simulink model "gm_IP_Core_SS_Switch_and_PWM"  (R2021a)
settings: Solver=VariableStepAuto  StartTime=0.0  StopTime=0.05  RelTol=1e-3
undefined symbols (not defined in the file or in its folder): f_FPGA_clk, T_FPGA_clk
libraries: hdlsllib x1
(part 2 of 2)

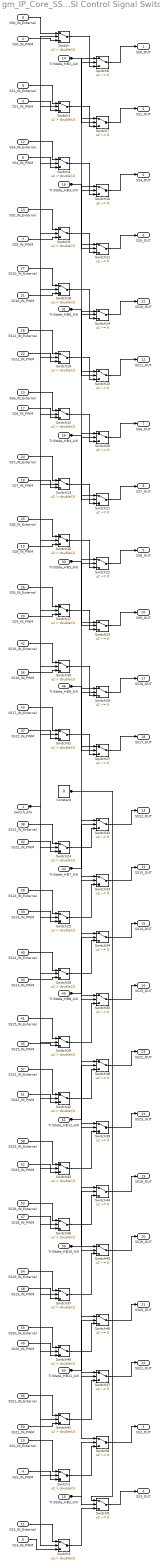
== system gm_IP_Core_SS_Switch_and_PWM/PWM_and_Switching_Signal_Control/VSI Control Signal Switch ==
  Switch_AXI : Inport  OutDataTypeStr=fixdt(0, 2, 0)  PortDimensions=1  SampleTime=1e-08
  SS0_IN_PWM : Inport  Port=2  OutDataTypeStr=fixdt(0, 1, 0)  PortDimensions=1  SampleTime=1e-08
  SS1_IN_PWM : Inport  Port=3  OutDataTypeStr=fixdt(0, 1, 0)  PortDimensions=1  SampleTime=1e-08
  SS2_IN_PWM : Inport  Port=4  OutDataTypeStr=fixdt(0, 1, 0)  PortDimensions=1  SampleTime=1e-08
  SS3_IN_PWM : Inport  Port=5  OutDataTypeStr=fixdt(0, 1, 0)  PortDimensions=1  SampleTime=1e-08
  SS4_IN_PWM : Inport  Port=6  OutDataTypeStr=fixdt(0, 1, 0)  PortDimensions=1  SampleTime=1e-08
  SS5_IN_PWM : Inport  Port=7  OutDataTypeStr=fixdt(0, 1, 0)  PortDimensions=1  SampleTime=1e-08
  SS0_IN_External : Inport  Port=8  OutDataTypeStr=boolean  PortDimensions=1  SampleTime=1e-08
  SS1_IN_External : Inport  Port=9  OutDataTypeStr=boolean  PortDimensions=1  SampleTime=1e-08
  SS2_IN_External : Inport  Port=10  OutDataTypeStr=boolean  PortDimensions=1  SampleTime=1e-08
  SS3_IN_External : Inport  Port=11  OutDataTypeStr=boolean  PortDimensions=1  SampleTime=1e-08
  SS4_IN_External : Inport  Port=12  OutDataTypeStr=boolean  PortDimensions=1  SampleTime=1e-08
  SS5_IN_External : Inport  Port=13  OutDataTypeStr=boolean  PortDimensions=1  SampleTime=1e-08
  TriState_HB1_AXI : Inport  Port=14  OutDataTypeStr=fixdt(0, 2, 0)  PortDimensions=1  SampleTime=1e-08
  TriState_HB2_AXI : Inport  Port=15  OutDataTypeStr=fixdt(0, 2, 0)  PortDimensions=1  SampleTime=1e-08
  TriState_HB3_AXI : Inport  Port=16  OutDataTypeStr=fixdt(0, 2, 0)  PortDimensions=1  SampleTime=1e-08
  SS6_IN_PWM : Inport  Port=17  OutDataTypeStr=fixdt(0, 1, 0)  PortDimensions=1  SampleTime=1e-08
  SS7_IN_PWM : Inport  Port=18  OutDataTypeStr=fixdt(0, 1, 0)  PortDimensions=1  SampleTime=1e-08
  SS8_IN_PWM : Inport  Port=19  OutDataTypeStr=fixdt(0, 1, 0)  PortDimensions=1  SampleTime=1e-08
  SS9_IN_PWM : Inport  Port=20  OutDataTypeStr=fixdt(0, 1, 0)  PortDimensions=1  SampleTime=1e-08
  SS10_IN_PWM : Inport  Port=21  OutDataTypeStr=fixdt(0, 1, 0)  PortDimensions=1  SampleTime=1e-08
  SS11_IN_PWM : Inport  Port=22  OutDataTypeStr=fixdt(0, 1, 0)  PortDimensions=1  SampleTime=1e-08
  SS6_IN_External : Inport  Port=23  OutDataTypeStr=boolean  PortDimensions=1  SampleTime=1e-08
  SS7_IN_External : Inport  Port=24  OutDataTypeStr=boolean  PortDimensions=1  SampleTime=1e-08
  SS8_IN_External : Inport  Port=25  OutDataTypeStr=boolean  PortDimensions=1  SampleTime=1e-08
  SS9_IN_External : Inport  Port=26  OutDataTypeStr=boolean  PortDimensions=1  SampleTime=1e-08
  SS10_IN_External : Inport  Port=27  OutDataTypeStr=boolean  PortDimensions=1  SampleTime=1e-08
  SS11_IN_External : Inport  Port=28  OutDataTypeStr=boolean  PortDimensions=1  SampleTime=1e-08
  TriState_HB4_AXI : Inport  Port=29  OutDataTypeStr=fixdt(0, 2, 0)  PortDimensions=1  SampleTime=1e-08
  TriState_HB5_AXI : Inport  Port=30  OutDataTypeStr=fixdt(0, 2, 0)  PortDimensions=1  SampleTime=1e-08
  TriState_HB6_AXI : Inport  Port=31  OutDataTypeStr=fixdt(0, 2, 0)  PortDimensions=1  SampleTime=1e-08
  SS12_IN_PWM : Inport  Port=32  OutDataTypeStr=fixdt(0, 1, 0)  PortDimensions=1  SampleTime=1e-08
  SS13_IN_PWM : Inport  Port=33  OutDataTypeStr=fixdt(0, 1, 0)  PortDimensions=1  SampleTime=1e-08
  SS14_IN_PWM : Inport  Port=34  OutDataTypeStr=fixdt(0, 1, 0)  PortDimensions=1  SampleTime=1e-08
  SS15_IN_PWM : Inport  Port=35  OutDataTypeStr=fixdt(0, 1, 0)  PortDimensions=1  SampleTime=1e-08
  SS16_IN_PWM : Inport  Port=36  OutDataTypeStr=fixdt(0, 1, 0)  PortDimensions=1  SampleTime=1e-08
  SS17_IN_PWM : Inport  Port=37  OutDataTypeStr=fixdt(0, 1, 0)  PortDimensions=1  SampleTime=1e-08
  SS12_IN_External : Inport  Port=38  OutDataTypeStr=boolean  PortDimensions=1  SampleTime=1e-08
  SS13_IN_External : Inport  Port=39  OutDataTypeStr=boolean  PortDimensions=1  SampleTime=1e-08
  SS14_IN_External : Inport  Port=40  OutDataTypeStr=boolean  PortDimensions=1  SampleTime=1e-08
  SS15_IN_External : Inport  Port=41  OutDataTypeStr=boolean  PortDimensions=1  SampleTime=1e-08
  SS16_IN_External : Inport  Port=42  OutDataTypeStr=boolean  PortDimensions=1  SampleTime=1e-08
  SS17_IN_External : Inport  Port=43  OutDataTypeStr=boolean  PortDimensions=1  SampleTime=1e-08
  TriState_HB7_AXI : Inport  Port=44  OutDataTypeStr=fixdt(0, 2, 0)  PortDimensions=1  SampleTime=1e-08
  TriState_HB8_AXI : Inport  Port=45  OutDataTypeStr=fixdt(0, 2, 0)  PortDimensions=1  SampleTime=1e-08
  TriState_HB9_AXI : Inport  Port=46  OutDataTypeStr=fixdt(0, 2, 0)  PortDimensions=1  SampleTime=1e-08
  SS18_IN_PWM : Inport  Port=47  OutDataTypeStr=fixdt(0, 1, 0)  PortDimensions=1  SampleTime=1e-08
  SS19_IN_PWM : Inport  Port=48  OutDataTypeStr=fixdt(0, 1, 0)  PortDimensions=1  SampleTime=1e-08
  SS20_IN_PWM : Inport  Port=49  OutDataTypeStr=fixdt(0, 1, 0)  PortDimensions=1  SampleTime=1e-08
  SS21_IN_PWM : Inport  Port=50  OutDataTypeStr=fixdt(0, 1, 0)  PortDimensions=1  SampleTime=1e-08
  SS22_IN_PWM : Inport  Port=51  OutDataTypeStr=fixdt(0, 1, 0)  PortDimensions=1  SampleTime=1e-08
  SS23_IN_PWM : Inport  Port=52  OutDataTypeStr=fixdt(0, 1, 0)  PortDimensions=1  SampleTime=1e-08
  SS18_IN_External : Inport  Port=53  OutDataTypeStr=boolean  PortDimensions=1  SampleTime=1e-08
  SS19_IN_External : Inport  Port=54  OutDataTypeStr=boolean  PortDimensions=1  SampleTime=1e-08
  SS20_IN_External : Inport  Port=55  OutDataTypeStr=boolean  PortDimensions=1  SampleTime=1e-08
  SS21_IN_External : Inport  Port=56  OutDataTypeStr=boolean  PortDimensions=1  SampleTime=1e-08
  SS22_IN_External : Inport  Port=57  OutDataTypeStr=boolean  PortDimensions=1  SampleTime=1e-08
  SS23_IN_External : Inport  Port=58  OutDataTypeStr=boolean  PortDimensions=1  SampleTime=1e-08
  TriState_HB10_AXI : Inport  Port=59  OutDataTypeStr=fixdt(0, 2, 0)  PortDimensions=1  SampleTime=1e-08
  TriState_HB11_AXI : Inport  Port=60  OutDataTypeStr=fixdt(0, 2, 0)  PortDimensions=1  SampleTime=1e-08
  TriState_HB12_AXI : Inport  Port=61  OutDataTypeStr=fixdt(0, 2, 0)  PortDimensions=1  SampleTime=1e-08
  Constant : Constant  Value=0  OutDataTypeStr=boolean  SampleTime=1e-08
  Switch{,1..5,12..13,16..19,24..25,28..31,36..37,40..43} (24 alike) : Switch  Criteria=u2 > Threshold  Threshold=double(1)  OutDataTypeStr=boolean  SampleTime=1e-08
  Switch{6..11,14..15,20..23,26..27,32..35,38..39,44..47} (24 alike) : Switch  Criteria=u2 ~= 0  Threshold=double(0)  OutDataTypeStr=boolean  SampleTime=1e-08
  SS0_OUT : Outport  SampleTime=1e-08  VectorParamsAs1DForOutWhenUnconnected=off
  SS1_OUT : Outport  Port=2  SampleTime=1e-08  VectorParamsAs1DForOutWhenUnconnected=off
  SS2_OUT : Outport  Port=3  SampleTime=1e-08  VectorParamsAs1DForOutWhenUnconnected=off
  SS3_OUT : Outport  Port=4  SampleTime=1e-08  VectorParamsAs1DForOutWhenUnconnected=off
  SS4_OUT : Outport  Port=5  SampleTime=1e-08  VectorParamsAs1DForOutWhenUnconnected=off
  SS5_OUT : Outport  Port=6  SampleTime=1e-08  VectorParamsAs1DForOutWhenUnconnected=off
  SS6_OUT : Outport  Port=7  SampleTime=1e-08  VectorParamsAs1DForOutWhenUnconnected=off
  SS7_OUT : Outport  Port=8  SampleTime=1e-08  VectorParamsAs1DForOutWhenUnconnected=off
  SS8_OUT : Outport  Port=9  SampleTime=1e-08  VectorParamsAs1DForOutWhenUnconnected=off
  SS9_OUT : Outport  Port=10  SampleTime=1e-08  VectorParamsAs1DForOutWhenUnconnected=off
  SS10_OUT : Outport  Port=11  SampleTime=1e-08  VectorParamsAs1DForOutWhenUnconnected=off
  SS11_OUT : Outport  Port=12  SampleTime=1e-08  VectorParamsAs1DForOutWhenUnconnected=off
  SS12_OUT : Outport  Port=13  SampleTime=1e-08  VectorParamsAs1DForOutWhenUnconnected=off
  SS13_OUT : Outport  Port=14  SampleTime=1e-08  VectorParamsAs1DForOutWhenUnconnected=off
  SS14_OUT : Outport  Port=15  SampleTime=1e-08  VectorParamsAs1DForOutWhenUnconnected=off
  SS15_OUT : Outport  Port=16  SampleTime=1e-08  VectorParamsAs1DForOutWhenUnconnected=off
  SS16_OUT : Outport  Port=17  SampleTime=1e-08  VectorParamsAs1DForOutWhenUnconnected=off
  SS17_OUT : Outport  Port=18  SampleTime=1e-08  VectorParamsAs1DForOutWhenUnconnected=off
  SS18_OUT : Outport  Port=19  SampleTime=1e-08  VectorParamsAs1DForOutWhenUnconnected=off
  SS19_OUT : Outport  Port=20  SampleTime=1e-08  VectorParamsAs1DForOutWhenUnconnected=off
  SS20_OUT : Outport  Port=21  SampleTime=1e-08  VectorParamsAs1DForOutWhenUnconnected=off
  SS21_OUT : Outport  Port=22  SampleTime=1e-08  VectorParamsAs1DForOutWhenUnconnected=off
  SS22_OUT : Outport  Port=23  SampleTime=1e-08  VectorParamsAs1DForOutWhenUnconnected=off
  SS23_OUT : Outport  Port=24  SampleTime=1e-08  VectorParamsAs1DForOutWhenUnconnected=off
  wires:
  Switch_AXI/1 -> Switch5/2, Switch43/2, Switch42/2, Switch41/2, Switch40/2, Switch4/2, Switch37/2, Switch36/2, Switch31/2, Switch30/2, Switch3/2, Switch29/2, Switch28/2, Switch25/2, Switch24/2, Switch2/2, Switch19/2, Switch18/2, Switch17/2, Switch16/2, Switch13/2, Switch12/2, Switch1/2, Switch/2
  SS0_IN_PWM/1 -> Switch/3
  SS1_IN_PWM/1 -> Switch1/3
  SS2_IN_PWM/1 -> Switch2/3
  SS3_IN_PWM/1 -> Switch3/3
  SS4_IN_PWM/1 -> Switch4/3
  SS5_IN_PWM/1 -> Switch5/3
  SS0_IN_External/1 -> Switch/1
  SS1_IN_External/1 -> Switch1/1
  SS2_IN_External/1 -> Switch2/1
  SS3_IN_External/1 -> Switch3/1
  SS4_IN_External/1 -> Switch4/1
  SS5_IN_External/1 -> Switch5/1
  TriState_HB1_AXI/1 -> Switch7/2, Switch6/2
  TriState_HB2_AXI/1 -> Switch9/2, Switch8/2
  TriState_HB3_AXI/1 -> Switch11/2, Switch10/2
  SS6_IN_PWM/1 -> Switch12/3
  SS7_IN_PWM/1 -> Switch13/3
  SS8_IN_PWM/1 -> Switch16/3
  SS9_IN_PWM/1 -> Switch17/3
  SS10_IN_PWM/1 -> Switch18/3
  SS11_IN_PWM/1 -> Switch19/3
  SS6_IN_External/1 -> Switch12/1
  SS7_IN_External/1 -> Switch13/1
  SS8_IN_External/1 -> Switch16/1
  SS9_IN_External/1 -> Switch17/1
  SS10_IN_External/1 -> Switch18/1
  SS11_IN_External/1 -> Switch19/1
  TriState_HB4_AXI/1 -> Switch21/2, Switch20/2
  TriState_HB5_AXI/1 -> Switch23/2, Switch22/2
  TriState_HB6_AXI/1 -> Switch15/2, Switch14/2
  SS12_IN_PWM/1 -> Switch24/3
  SS13_IN_PWM/1 -> Switch25/3
  SS14_IN_PWM/1 -> Switch28/3
  SS15_IN_PWM/1 -> Switch29/3
  SS16_IN_PWM/1 -> Switch30/3
  SS17_IN_PWM/1 -> Switch31/3
  SS12_IN_External/1 -> Switch24/1
  SS13_IN_External/1 -> Switch25/1
  SS14_IN_External/1 -> Switch28/1
  SS15_IN_External/1 -> Switch29/1
  SS16_IN_External/1 -> Switch30/1
  SS17_IN_External/1 -> Switch31/1
  TriState_HB7_AXI/1 -> Switch33/2, Switch32/2
  TriState_HB8_AXI/1 -> Switch35/2, Switch34/2
  TriState_HB9_AXI/1 -> Switch27/2, Switch26/2
  SS18_IN_PWM/1 -> Switch36/3
  SS19_IN_PWM/1 -> Switch37/3
  SS20_IN_PWM/1 -> Switch40/3
  SS21_IN_PWM/1 -> Switch41/3
  SS22_IN_PWM/1 -> Switch42/3
  SS23_IN_PWM/1 -> Switch43/3
  SS18_IN_External/1 -> Switch36/1
  SS19_IN_External/1 -> Switch37/1
  SS20_IN_External/1 -> Switch40/1
  SS21_IN_External/1 -> Switch41/1
  SS22_IN_External/1 -> Switch42/1
  SS23_IN_External/1 -> Switch43/1
  TriState_HB10_AXI/1 -> Switch45/2, Switch44/2
  TriState_HB11_AXI/1 -> Switch47/2, Switch46/2
  TriState_HB12_AXI/1 -> Switch39/2, Switch38/2
  Constant/1 -> Switch9/1, Switch8/1, Switch7/1, Switch6/1, Switch47/1, Switch46/1, Switch45/1, Switch44/1, Switch39/1, Switch38/1, Switch35/1, Switch34/1, Switch33/1, Switch32/1, Switch27/1, Switch26/1, Switch23/1, Switch22/1, Switch21/1, Switch20/1, Switch15/1, Switch14/1, Switch11/1, Switch10/1
  Switch/1 -> Switch6/3
  Switch1/1 -> Switch7/3
  Switch10/1 -> SS4_OUT/1
  Switch11/1 -> SS5_OUT/1
  Switch12/1 -> Switch20/3
  Switch13/1 -> Switch21/3
  Switch14/1 -> SS10_OUT/1
  Switch15/1 -> SS11_OUT/1
  Switch16/1 -> Switch22/3
  Switch17/1 -> Switch23/3
  Switch18/1 -> Switch14/3
  Switch19/1 -> Switch15/3
  Switch2/1 -> Switch8/3
  Switch20/1 -> SS6_OUT/1
  Switch21/1 -> SS7_OUT/1
  Switch22/1 -> SS8_OUT/1
  Switch23/1 -> SS9_OUT/1
  Switch24/1 -> Switch32/3
  Switch25/1 -> Switch33/3
  Switch26/1 -> SS16_OUT/1
  Switch27/1 -> SS17_OUT/1
  Switch28/1 -> Switch34/3
  Switch29/1 -> Switch35/3
  Switch3/1 -> Switch9/3
  Switch30/1 -> Switch26/3
  Switch31/1 -> Switch27/3
  Switch32/1 -> SS12_OUT/1
  Switch33/1 -> SS13_OUT/1
  Switch34/1 -> SS14_OUT/1
  Switch35/1 -> SS15_OUT/1
  Switch36/1 -> Switch44/3
  Switch37/1 -> Switch45/3
  Switch38/1 -> SS22_OUT/1
  Switch39/1 -> SS23_OUT/1
  Switch4/1 -> Switch10/3
  Switch40/1 -> Switch46/3
  Switch41/1 -> Switch47/3
  Switch42/1 -> Switch38/3
  Switch43/1 -> Switch39/3
  Switch44/1 -> SS18_OUT/1
  Switch45/1 -> SS19_OUT/1
  Switch46/1 -> SS20_OUT/1
  Switch47/1 -> SS21_OUT/1
  Switch5/1 -> Switch11/3
  Switch6/1 -> SS0_OUT/1
  Switch7/1 -> SS1_OUT/1
  Switch8/1 -> SS2_OUT/1
  Switch9/1 -> SS3_OUT/1

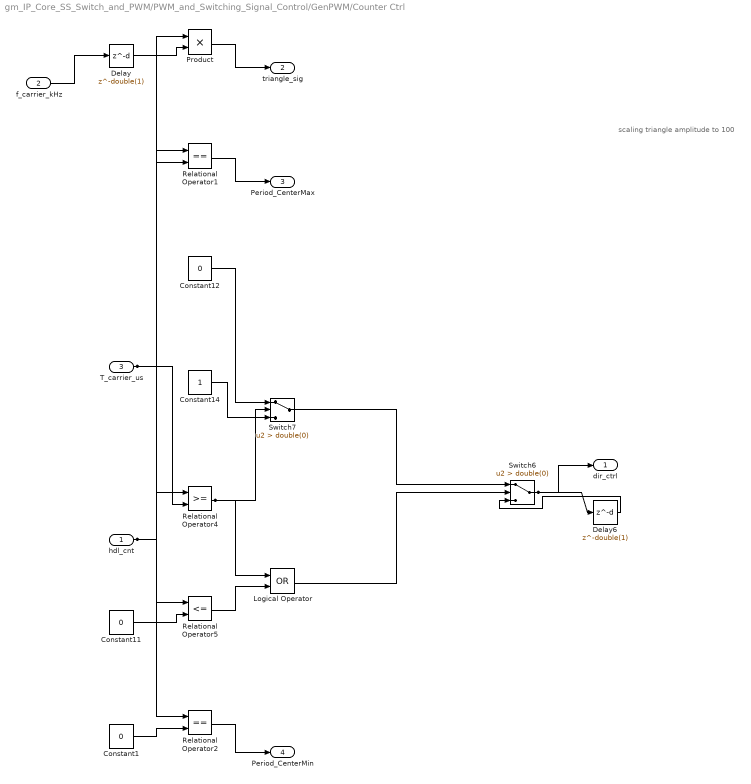
== system gm_IP_Core_SS_Switch_and_PWM/PWM_and_Switching_Signal_Control/GenPWM/Counter Ctrl ==
  note: scaling triangle amplitude to 100
  hdl_cnt : Inport  OutDataTypeStr=fixdt(0, 20, 0)  PortDimensions=1  SampleTime=1e-08
  f_carrier_kHz : Inport  Port=2  OutDataTypeStr=fixdt(0, 25, 26)  PortDimensions=1  SampleTime=1e-08
  T_carrier_us : Inport  Port=3  OutDataTypeStr=fixdt(0, 25, 0)  PortDimensions=1  SampleTime=1e-08
  Constant1 : Constant  Value=0  OutDataTypeStr=fixdt(0, 20, 0)  SampleTime=1e-08
  Constant11 : Constant  Value=0  OutDataTypeStr=fixdt(0, 20, 0)  SampleTime=1e-08
  Constant12 : Constant  Value=0  OutDataTypeStr=boolean  SampleTime=1e-08
  Constant14 : Constant  OutDataTypeStr=boolean  SampleTime=1e-08
  Delay : Delay  DelayLength=double(1)  InitialCondition=0  SampleTime=1e-08
  Delay6 : Delay  DelayLength=double(1)  InitialCondition=0  SampleTime=1e-08
  Logical Operator : Logic  Operator=OR  AllPortsSameDT=off  OutDataTypeStr=boolean  SampleTime=1e-08
  Product : Product  Inputs=**  OutDataTypeStr=fixdt(0, 18, 17)  SampleTime=1e-08
  Relational Operator1 : RelationalOperator  Operator===  OutDataTypeStr=boolean  SampleTime=1e-08  RndMeth=Nearest
  Relational Operator2 : RelationalOperator  Operator===  OutDataTypeStr=boolean  SampleTime=1e-08  RndMeth=Nearest
  Relational Operator4 : RelationalOperator  OutDataTypeStr=boolean  SampleTime=1e-08  RndMeth=Nearest
  Relational Operator5 : RelationalOperator  Operator=<=  OutDataTypeStr=boolean  SampleTime=1e-08  RndMeth=Nearest
  Switch6 : Switch  Criteria=u2 > Threshold  Threshold=double(0)  OutDataTypeStr=boolean  SampleTime=1e-08
  Switch7 : Switch  Criteria=u2 > Threshold  Threshold=double(0)  OutDataTypeStr=boolean  SampleTime=1e-08
  dir_ctrl : Outport  SampleTime=1e-08  VectorParamsAs1DForOutWhenUnconnected=off
  triangle_sig : Outport  Port=2  SampleTime=1e-08  VectorParamsAs1DForOutWhenUnconnected=off
  Period_CenterMax : Outport  Port=3  SampleTime=1e-08  VectorParamsAs1DForOutWhenUnconnected=off
  Period_CenterMin : Outport  Port=4  SampleTime=1e-08  VectorParamsAs1DForOutWhenUnconnected=off
  wires:
  hdl_cnt/1 -> Relational Operator5/1, Relational Operator4/1, Relational Operator2/1, Relational Operator1/1, Product/1
  f_carrier_kHz/1 -> Delay/1
  T_carrier_us/1 -> Relational Operator4/2, Relational Operator1/2
  Constant1/1 -> Relational Operator2/2
  Constant11/1 -> Relational Operator5/2
  Constant12/1 -> Switch7/1
  Constant14/1 -> Switch7/3
  Delay/1 -> Product/2
  Delay6/1 -> Switch6/3
  Logical Operator/1 -> Switch6/2
  Product/1 -> triangle_sig/1
  Relational Operator1/1 -> Period_CenterMax/1
  Relational Operator2/1 -> Period_CenterMin/1
  Relational Operator4/1 -> Switch7/2, Logical Operator/1
  Relational Operator5/1 -> Logical Operator/2
  Switch6/1 -> Delay6/1, dir_ctrl/1
  Switch7/1 -> Switch6/1

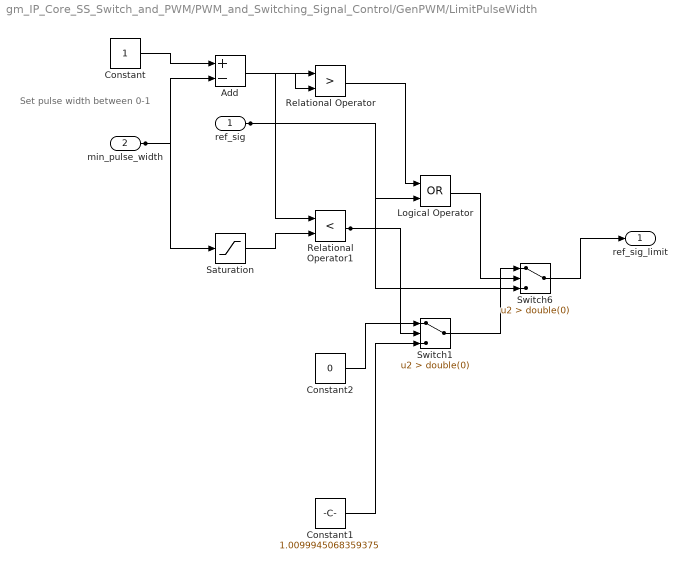
== system gm_IP_Core_SS_Switch_and_PWM/PWM_and_Switching_Signal_Control/GenPWM/LimitPulseWidth ==
  note: Set pulse width between 0-1
  ref_sig : Inport  OutDataTypeStr=fixdt(1, 14, 12)  PortDimensions=1  SampleTime=1e-08
  min_pulse_width : Inport  Port=2  OutDataTypeStr=fixdt(1, 18, 16)  PortDimensions=1  SampleTime=1e-08
  Add : Sum  Inputs=+-  AccumDataTypeStr=fixdt(1, 19, 16)  OutDataTypeStr=fixdt(1, 18, 16)  SampleTime=1e-08
  Constant : Constant  OutDataTypeStr=fixdt(1, 18, 16)  SampleTime=1e-08
  Constant1 : Constant  Value=1.0099945068359375  OutDataTypeStr=fixdt(1, 18, 16)  SampleTime=1e-08
  Constant2 : Constant  Value=0  OutDataTypeStr=fixdt(1, 18, 16)  SampleTime=1e-08
  Logical Operator : Logic  Operator=OR  AllPortsSameDT=off  OutDataTypeStr=boolean  SampleTime=1e-08
  Relational Operator : RelationalOperator  Operator=>  OutDataTypeStr=boolean  SampleTime=1e-08  RndMeth=Nearest
  Relational Operator1 : RelationalOperator  Operator=<  OutDataTypeStr=boolean  SampleTime=1e-08  RndMeth=Nearest
  Saturation : Saturate  UpperLimit="fi(0,1,18,16,\"hex\",\"10000\")"  LowerLimit="fi(0,1,18,16,\"hex\",\"00000\")"  SampleTime=1e-08  OutDataTypeStr=fixdt(1, 18, 16)
  Switch1 : Switch  Criteria=u2 > Threshold  Threshold=double(0)  OutDataTypeStr=fixdt(1, 18, 16)  SampleTime=1e-08
  Switch6 : Switch  Criteria=u2 > Threshold  Threshold=double(0)  OutDataTypeStr=fixdt(1, 18, 16)  SampleTime=1e-08
  ref_sig_limit : Outport  SampleTime=1e-08  VectorParamsAs1DForOutWhenUnconnected=off
  wires:
  ref_sig/1 -> Switch6/3, Relational Operator1/1, Relational Operator/1
  min_pulse_width/1 -> Saturation/1, Add/2
  Add/1 -> Relational Operator/2
  Constant/1 -> Add/1
  Constant1/1 -> Switch1/3
  Constant2/1 -> Switch1/1
  Logical Operator/1 -> Switch6/2
  Relational Operator/1 -> Logical Operator/1
  Relational Operator1/1 -> Switch1/2, Logical Operator/2
  Saturation/1 -> Relational Operator1/2
  Switch1/1 -> Switch6/1
  Switch6/1 -> ref_sig_limit/1

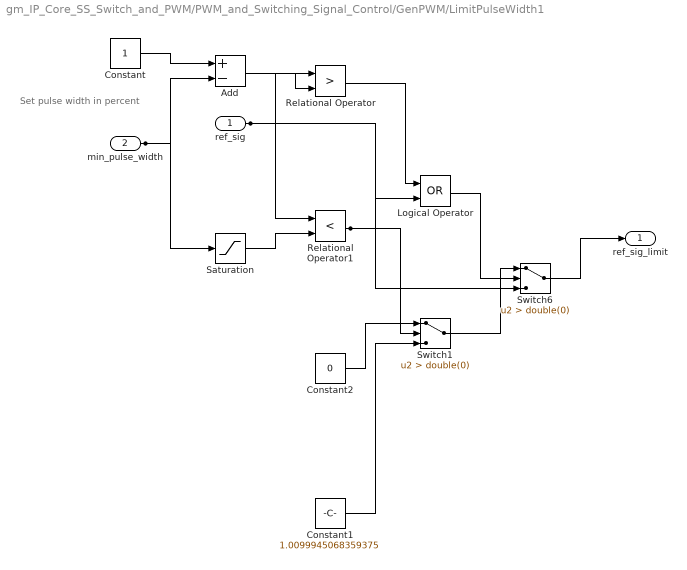
== system gm_IP_Core_SS_Switch_and_PWM/PWM_and_Switching_Signal_Control/GenPWM/LimitPulseWidth1 ==
  note: Set pulse width in percent
  ref_sig : Inport  OutDataTypeStr=fixdt(1, 14, 12)  PortDimensions=1  SampleTime=1e-08
  min_pulse_width : Inport  Port=2  OutDataTypeStr=fixdt(1, 18, 16)  PortDimensions=1  SampleTime=1e-08
  Add : Sum  Inputs=+-  AccumDataTypeStr=fixdt(1, 19, 16)  OutDataTypeStr=fixdt(1, 18, 16)  SampleTime=1e-08
  Constant : Constant  OutDataTypeStr=fixdt(1, 18, 16)  SampleTime=1e-08
  Constant1 : Constant  Value=1.0099945068359375  OutDataTypeStr=fixdt(1, 18, 16)  SampleTime=1e-08
  Constant2 : Constant  Value=0  OutDataTypeStr=fixdt(1, 18, 16)  SampleTime=1e-08
  Logical Operator : Logic  Operator=OR  AllPortsSameDT=off  OutDataTypeStr=boolean  SampleTime=1e-08
  Relational Operator : RelationalOperator  Operator=>  OutDataTypeStr=boolean  SampleTime=1e-08  RndMeth=Nearest
  Relational Operator1 : RelationalOperator  Operator=<  OutDataTypeStr=boolean  SampleTime=1e-08  RndMeth=Nearest
  Saturation : Saturate  UpperLimit="fi(0,1,18,16,\"hex\",\"10000\")"  LowerLimit="fi(0,1,18,16,\"hex\",\"00000\")"  SampleTime=1e-08  OutDataTypeStr=fixdt(1, 18, 16)
  Switch1 : Switch  Criteria=u2 > Threshold  Threshold=double(0)  OutDataTypeStr=fixdt(1, 18, 16)  SampleTime=1e-08
  Switch6 : Switch  Criteria=u2 > Threshold  Threshold=double(0)  OutDataTypeStr=fixdt(1, 18, 16)  SampleTime=1e-08
  ref_sig_limit : Outport  SampleTime=1e-08  VectorParamsAs1DForOutWhenUnconnected=off
  wires:
  ref_sig/1 -> Switch6/3, Relational Operator1/1, Relational Operator/1
  min_pulse_width/1 -> Saturation/1, Add/2
  Add/1 -> Relational Operator/2
  Constant/1 -> Add/1
  Constant1/1 -> Switch1/3
  Constant2/1 -> Switch1/1
  Logical Operator/1 -> Switch6/2
  Relational Operator/1 -> Logical Operator/1
  Relational Operator1/1 -> Switch1/2, Logical Operator/2
  Saturation/1 -> Relational Operator1/2
  Switch1/1 -> Switch6/1
  Switch6/1 -> ref_sig_limit/1

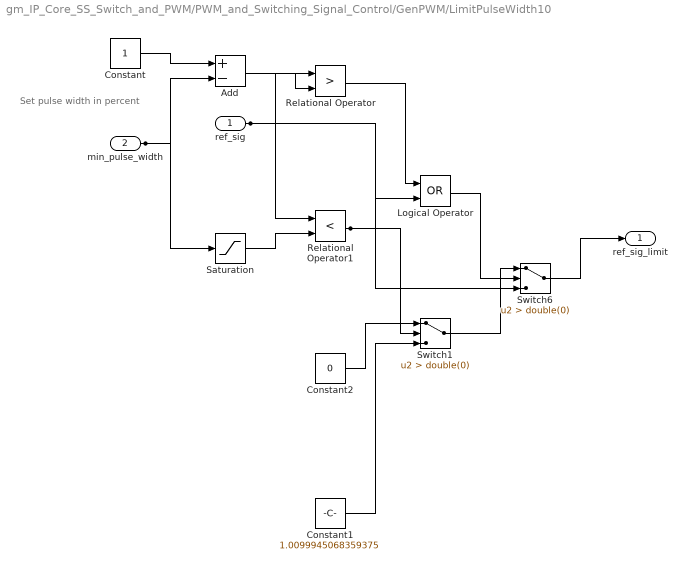
== system gm_IP_Core_SS_Switch_and_PWM/PWM_and_Switching_Signal_Control/GenPWM/LimitPulseWidth10 ==
  note: Set pulse width in percent
  ref_sig : Inport  OutDataTypeStr=fixdt(1, 14, 12)  PortDimensions=1  SampleTime=1e-08
  min_pulse_width : Inport  Port=2  OutDataTypeStr=fixdt(1, 18, 16)  PortDimensions=1  SampleTime=1e-08
  Add : Sum  Inputs=+-  AccumDataTypeStr=fixdt(1, 19, 16)  OutDataTypeStr=fixdt(1, 18, 16)  SampleTime=1e-08
  Constant : Constant  OutDataTypeStr=fixdt(1, 18, 16)  SampleTime=1e-08
  Constant1 : Constant  Value=1.0099945068359375  OutDataTypeStr=fixdt(1, 18, 16)  SampleTime=1e-08
  Constant2 : Constant  Value=0  OutDataTypeStr=fixdt(1, 18, 16)  SampleTime=1e-08
  Logical Operator : Logic  Operator=OR  AllPortsSameDT=off  OutDataTypeStr=boolean  SampleTime=1e-08
  Relational Operator : RelationalOperator  Operator=>  OutDataTypeStr=boolean  SampleTime=1e-08  RndMeth=Nearest
  Relational Operator1 : RelationalOperator  Operator=<  OutDataTypeStr=boolean  SampleTime=1e-08  RndMeth=Nearest
  Saturation : Saturate  UpperLimit="fi(0,1,18,16,\"hex\",\"10000\")"  LowerLimit="fi(0,1,18,16,\"hex\",\"00000\")"  SampleTime=1e-08  OutDataTypeStr=fixdt(1, 18, 16)
  Switch1 : Switch  Criteria=u2 > Threshold  Threshold=double(0)  OutDataTypeStr=fixdt(1, 18, 16)  SampleTime=1e-08
  Switch6 : Switch  Criteria=u2 > Threshold  Threshold=double(0)  OutDataTypeStr=fixdt(1, 18, 16)  SampleTime=1e-08
  ref_sig_limit : Outport  SampleTime=1e-08  VectorParamsAs1DForOutWhenUnconnected=off
  wires:
  ref_sig/1 -> Switch6/3, Relational Operator1/1, Relational Operator/1
  min_pulse_width/1 -> Saturation/1, Add/2
  Add/1 -> Relational Operator/2
  Constant/1 -> Add/1
  Constant1/1 -> Switch1/3
  Constant2/1 -> Switch1/1
  Logical Operator/1 -> Switch6/2
  Relational Operator/1 -> Logical Operator/1
  Relational Operator1/1 -> Switch1/2, Logical Operator/2
  Saturation/1 -> Relational Operator1/2
  Switch1/1 -> Switch6/1
  Switch6/1 -> ref_sig_limit/1

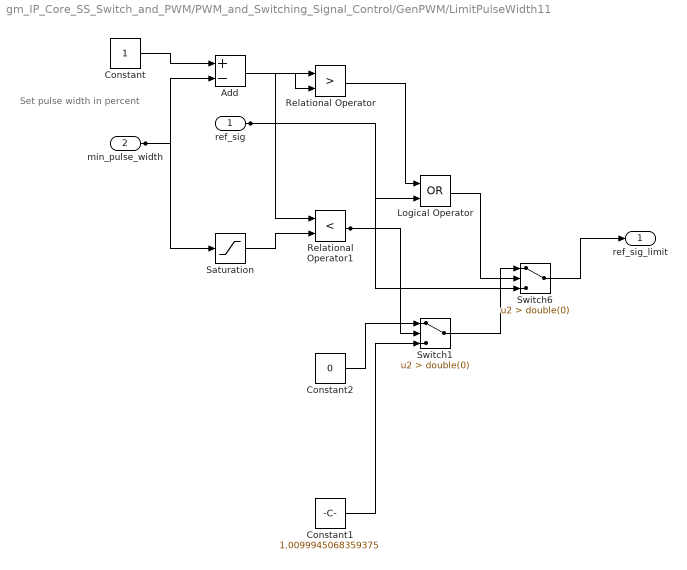
== system gm_IP_Core_SS_Switch_and_PWM/PWM_and_Switching_Signal_Control/GenPWM/LimitPulseWidth11 ==
  note: Set pulse width in percent
  ref_sig : Inport  OutDataTypeStr=fixdt(1, 14, 12)  PortDimensions=1  SampleTime=1e-08
  min_pulse_width : Inport  Port=2  OutDataTypeStr=fixdt(1, 18, 16)  PortDimensions=1  SampleTime=1e-08
  Add : Sum  Inputs=+-  AccumDataTypeStr=fixdt(1, 19, 16)  OutDataTypeStr=fixdt(1, 18, 16)  SampleTime=1e-08
  Constant : Constant  OutDataTypeStr=fixdt(1, 18, 16)  SampleTime=1e-08
  Constant1 : Constant  Value=1.0099945068359375  OutDataTypeStr=fixdt(1, 18, 16)  SampleTime=1e-08
  Constant2 : Constant  Value=0  OutDataTypeStr=fixdt(1, 18, 16)  SampleTime=1e-08
  Logical Operator : Logic  Operator=OR  AllPortsSameDT=off  OutDataTypeStr=boolean  SampleTime=1e-08
  Relational Operator : RelationalOperator  Operator=>  OutDataTypeStr=boolean  SampleTime=1e-08  RndMeth=Nearest
  Relational Operator1 : RelationalOperator  Operator=<  OutDataTypeStr=boolean  SampleTime=1e-08  RndMeth=Nearest
  Saturation : Saturate  UpperLimit="fi(0,1,18,16,\"hex\",\"10000\")"  LowerLimit="fi(0,1,18,16,\"hex\",\"00000\")"  SampleTime=1e-08  OutDataTypeStr=fixdt(1, 18, 16)
  Switch1 : Switch  Criteria=u2 > Threshold  Threshold=double(0)  OutDataTypeStr=fixdt(1, 18, 16)  SampleTime=1e-08
  Switch6 : Switch  Criteria=u2 > Threshold  Threshold=double(0)  OutDataTypeStr=fixdt(1, 18, 16)  SampleTime=1e-08
  ref_sig_limit : Outport  SampleTime=1e-08  VectorParamsAs1DForOutWhenUnconnected=off
  wires:
  ref_sig/1 -> Switch6/3, Relational Operator1/1, Relational Operator/1
  min_pulse_width/1 -> Saturation/1, Add/2
  Add/1 -> Relational Operator/2
  Constant/1 -> Add/1
  Constant1/1 -> Switch1/3
  Constant2/1 -> Switch1/1
  Logical Operator/1 -> Switch6/2
  Relational Operator/1 -> Logical Operator/1
  Relational Operator1/1 -> Switch1/2, Logical Operator/2
  Saturation/1 -> Relational Operator1/2
  Switch1/1 -> Switch6/1
  Switch6/1 -> ref_sig_limit/1

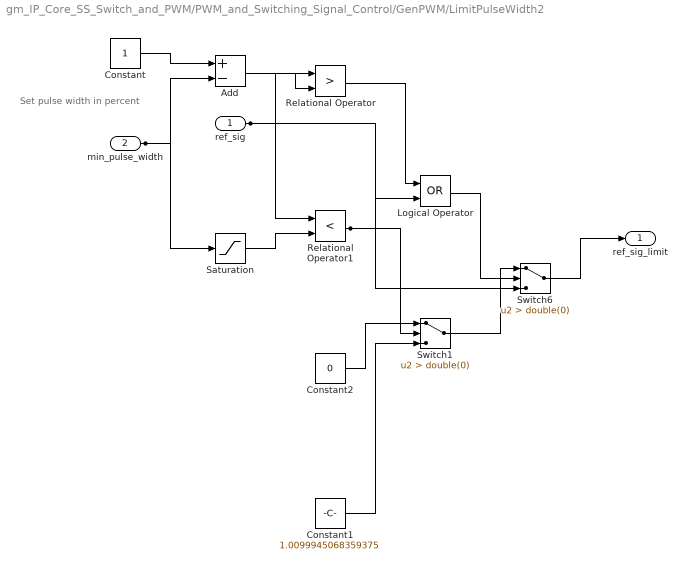
== system gm_IP_Core_SS_Switch_and_PWM/PWM_and_Switching_Signal_Control/GenPWM/LimitPulseWidth2 ==
  note: Set pulse width in percent
  ref_sig : Inport  OutDataTypeStr=fixdt(1, 14, 12)  PortDimensions=1  SampleTime=1e-08
  min_pulse_width : Inport  Port=2  OutDataTypeStr=fixdt(1, 18, 16)  PortDimensions=1  SampleTime=1e-08
  Add : Sum  Inputs=+-  AccumDataTypeStr=fixdt(1, 19, 16)  OutDataTypeStr=fixdt(1, 18, 16)  SampleTime=1e-08
  Constant : Constant  OutDataTypeStr=fixdt(1, 18, 16)  SampleTime=1e-08
  Constant1 : Constant  Value=1.0099945068359375  OutDataTypeStr=fixdt(1, 18, 16)  SampleTime=1e-08
  Constant2 : Constant  Value=0  OutDataTypeStr=fixdt(1, 18, 16)  SampleTime=1e-08
  Logical Operator : Logic  Operator=OR  AllPortsSameDT=off  OutDataTypeStr=boolean  SampleTime=1e-08
  Relational Operator : RelationalOperator  Operator=>  OutDataTypeStr=boolean  SampleTime=1e-08  RndMeth=Nearest
  Relational Operator1 : RelationalOperator  Operator=<  OutDataTypeStr=boolean  SampleTime=1e-08  RndMeth=Nearest
  Saturation : Saturate  UpperLimit="fi(0,1,18,16,\"hex\",\"10000\")"  LowerLimit="fi(0,1,18,16,\"hex\",\"00000\")"  SampleTime=1e-08  OutDataTypeStr=fixdt(1, 18, 16)
  Switch1 : Switch  Criteria=u2 > Threshold  Threshold=double(0)  OutDataTypeStr=fixdt(1, 18, 16)  SampleTime=1e-08
  Switch6 : Switch  Criteria=u2 > Threshold  Threshold=double(0)  OutDataTypeStr=fixdt(1, 18, 16)  SampleTime=1e-08
  ref_sig_limit : Outport  SampleTime=1e-08  VectorParamsAs1DForOutWhenUnconnected=off
  wires:
  ref_sig/1 -> Switch6/3, Relational Operator1/1, Relational Operator/1
  min_pulse_width/1 -> Saturation/1, Add/2
  Add/1 -> Relational Operator/2
  Constant/1 -> Add/1
  Constant1/1 -> Switch1/3
  Constant2/1 -> Switch1/1
  Logical Operator/1 -> Switch6/2
  Relational Operator/1 -> Logical Operator/1
  Relational Operator1/1 -> Switch1/2, Logical Operator/2
  Saturation/1 -> Relational Operator1/2
  Switch1/1 -> Switch6/1
  Switch6/1 -> ref_sig_limit/1

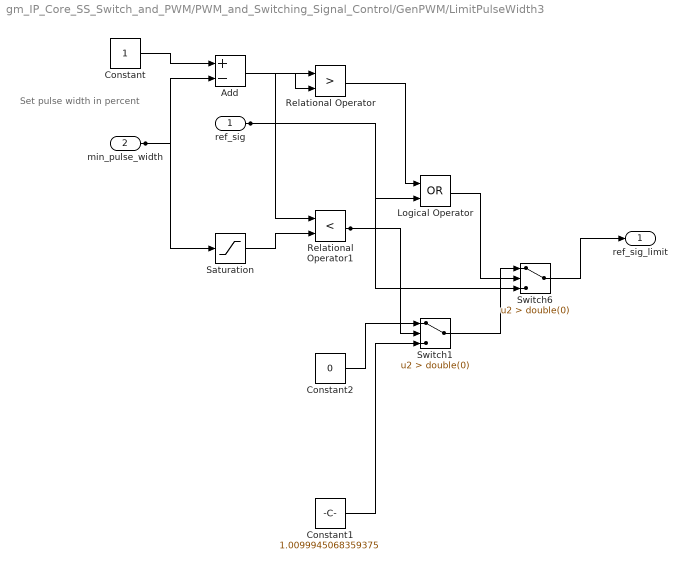
== system gm_IP_Core_SS_Switch_and_PWM/PWM_and_Switching_Signal_Control/GenPWM/LimitPulseWidth3 ==
  note: Set pulse width in percent
  ref_sig : Inport  OutDataTypeStr=fixdt(1, 14, 12)  PortDimensions=1  SampleTime=1e-08
  min_pulse_width : Inport  Port=2  OutDataTypeStr=fixdt(1, 18, 16)  PortDimensions=1  SampleTime=1e-08
  Add : Sum  Inputs=+-  AccumDataTypeStr=fixdt(1, 19, 16)  OutDataTypeStr=fixdt(1, 18, 16)  SampleTime=1e-08
  Constant : Constant  OutDataTypeStr=fixdt(1, 18, 16)  SampleTime=1e-08
  Constant1 : Constant  Value=1.0099945068359375  OutDataTypeStr=fixdt(1, 18, 16)  SampleTime=1e-08
  Constant2 : Constant  Value=0  OutDataTypeStr=fixdt(1, 18, 16)  SampleTime=1e-08
  Logical Operator : Logic  Operator=OR  AllPortsSameDT=off  OutDataTypeStr=boolean  SampleTime=1e-08
  Relational Operator : RelationalOperator  Operator=>  OutDataTypeStr=boolean  SampleTime=1e-08  RndMeth=Nearest
  Relational Operator1 : RelationalOperator  Operator=<  OutDataTypeStr=boolean  SampleTime=1e-08  RndMeth=Nearest
  Saturation : Saturate  UpperLimit="fi(0,1,18,16,\"hex\",\"10000\")"  LowerLimit="fi(0,1,18,16,\"hex\",\"00000\")"  SampleTime=1e-08  OutDataTypeStr=fixdt(1, 18, 16)
  Switch1 : Switch  Criteria=u2 > Threshold  Threshold=double(0)  OutDataTypeStr=fixdt(1, 18, 16)  SampleTime=1e-08
  Switch6 : Switch  Criteria=u2 > Threshold  Threshold=double(0)  OutDataTypeStr=fixdt(1, 18, 16)  SampleTime=1e-08
  ref_sig_limit : Outport  SampleTime=1e-08  VectorParamsAs1DForOutWhenUnconnected=off
  wires:
  ref_sig/1 -> Switch6/3, Relational Operator1/1, Relational Operator/1
  min_pulse_width/1 -> Saturation/1, Add/2
  Add/1 -> Relational Operator/2
  Constant/1 -> Add/1
  Constant1/1 -> Switch1/3
  Constant2/1 -> Switch1/1
  Logical Operator/1 -> Switch6/2
  Relational Operator/1 -> Logical Operator/1
  Relational Operator1/1 -> Switch1/2, Logical Operator/2
  Saturation/1 -> Relational Operator1/2
  Switch1/1 -> Switch6/1
  Switch6/1 -> ref_sig_limit/1

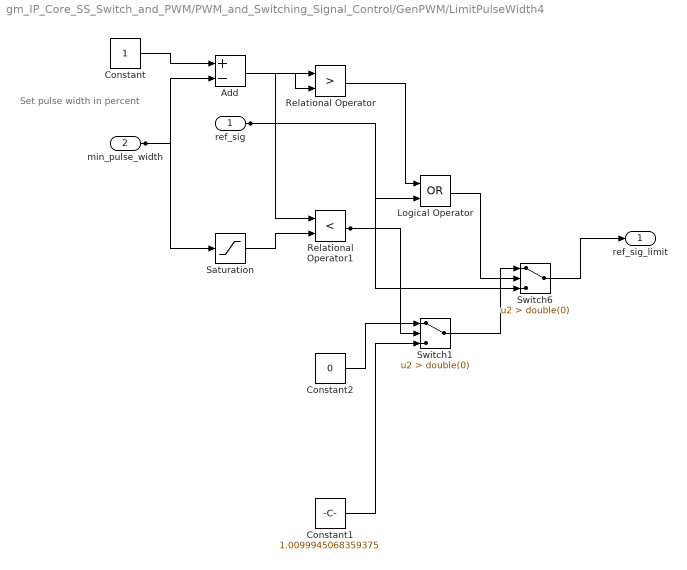
== system gm_IP_Core_SS_Switch_and_PWM/PWM_and_Switching_Signal_Control/GenPWM/LimitPulseWidth4 ==
  note: Set pulse width in percent
  ref_sig : Inport  OutDataTypeStr=fixdt(1, 14, 12)  PortDimensions=1  SampleTime=1e-08
  min_pulse_width : Inport  Port=2  OutDataTypeStr=fixdt(1, 18, 16)  PortDimensions=1  SampleTime=1e-08
  Add : Sum  Inputs=+-  AccumDataTypeStr=fixdt(1, 19, 16)  OutDataTypeStr=fixdt(1, 18, 16)  SampleTime=1e-08
  Constant : Constant  OutDataTypeStr=fixdt(1, 18, 16)  SampleTime=1e-08
  Constant1 : Constant  Value=1.0099945068359375  OutDataTypeStr=fixdt(1, 18, 16)  SampleTime=1e-08
  Constant2 : Constant  Value=0  OutDataTypeStr=fixdt(1, 18, 16)  SampleTime=1e-08
  Logical Operator : Logic  Operator=OR  AllPortsSameDT=off  OutDataTypeStr=boolean  SampleTime=1e-08
  Relational Operator : RelationalOperator  Operator=>  OutDataTypeStr=boolean  SampleTime=1e-08  RndMeth=Nearest
  Relational Operator1 : RelationalOperator  Operator=<  OutDataTypeStr=boolean  SampleTime=1e-08  RndMeth=Nearest
  Saturation : Saturate  UpperLimit="fi(0,1,18,16,\"hex\",\"10000\")"  LowerLimit="fi(0,1,18,16,\"hex\",\"00000\")"  SampleTime=1e-08  OutDataTypeStr=fixdt(1, 18, 16)
  Switch1 : Switch  Criteria=u2 > Threshold  Threshold=double(0)  OutDataTypeStr=fixdt(1, 18, 16)  SampleTime=1e-08
  Switch6 : Switch  Criteria=u2 > Threshold  Threshold=double(0)  OutDataTypeStr=fixdt(1, 18, 16)  SampleTime=1e-08
  ref_sig_limit : Outport  SampleTime=1e-08  VectorParamsAs1DForOutWhenUnconnected=off
  wires:
  ref_sig/1 -> Switch6/3, Relational Operator1/1, Relational Operator/1
  min_pulse_width/1 -> Saturation/1, Add/2
  Add/1 -> Relational Operator/2
  Constant/1 -> Add/1
  Constant1/1 -> Switch1/3
  Constant2/1 -> Switch1/1
  Logical Operator/1 -> Switch6/2
  Relational Operator/1 -> Logical Operator/1
  Relational Operator1/1 -> Switch1/2, Logical Operator/2
  Saturation/1 -> Relational Operator1/2
  Switch1/1 -> Switch6/1
  Switch6/1 -> ref_sig_limit/1

== system gm_IP_Core_SS_Switch_and_PWM/PWM_and_Switching_Signal_Control/GenPWM/LimitPulseWidth5 ==
  note: Set pulse width in percent
  ref_sig : Inport  OutDataTypeStr=fixdt(1, 14, 12)  PortDimensions=1  SampleTime=1e-08
  min_pulse_width : Inport  Port=2  OutDataTypeStr=fixdt(1, 18, 16)  PortDimensions=1  SampleTime=1e-08
  Add : Sum  Inputs=+-  AccumDataTypeStr=fixdt(1, 19, 16)  OutDataTypeStr=fixdt(1, 18, 16)  SampleTime=1e-08
  Constant : Constant  OutDataTypeStr=fixdt(1, 18, 16)  SampleTime=1e-08
  Constant1 : Constant  Value=1.0099945068359375  OutDataTypeStr=fixdt(1, 18, 16)  SampleTime=1e-08
  Constant2 : Constant  Value=0  OutDataTypeStr=fixdt(1, 18, 16)  SampleTime=1e-08
  Logical Operator : Logic  Operator=OR  AllPortsSameDT=off  OutDataTypeStr=boolean  SampleTime=1e-08
  Relational Operator : RelationalOperator  Operator=>  OutDataTypeStr=boolean  SampleTime=1e-08  RndMeth=Nearest
  Relational Operator1 : RelationalOperator  Operator=<  OutDataTypeStr=boolean  SampleTime=1e-08  RndMeth=Nearest
  Saturation : Saturate  UpperLimit="fi(0,1,18,16,\"hex\",\"10000\")"  LowerLimit="fi(0,1,18,16,\"hex\",\"00000\")"  SampleTime=1e-08  OutDataTypeStr=fixdt(1, 18, 16)
  Switch1 : Switch  Criteria=u2 > Threshold  Threshold=double(0)  OutDataTypeStr=fixdt(1, 18, 16)  SampleTime=1e-08
  Switch6 : Switch  Criteria=u2 > Threshold  Threshold=double(0)  OutDataTypeStr=fixdt(1, 18, 16)  SampleTime=1e-08
  ref_sig_limit : Outport  SampleTime=1e-08  VectorParamsAs1DForOutWhenUnconnected=off
  wires:
  ref_sig/1 -> Switch6/3, Relational Operator1/1, Relational Operator/1
  min_pulse_width/1 -> Saturation/1, Add/2
  Add/1 -> Relational Operator/2
  Constant/1 -> Add/1
  Constant1/1 -> Switch1/3
  Constant2/1 -> Switch1/1
  Logical Operator/1 -> Switch6/2
  Relational Operator/1 -> Logical Operator/1
  Relational Operator1/1 -> Switch1/2, Logical Operator/2
  Saturation/1 -> Relational Operator1/2
  Switch1/1 -> Switch6/1
  Switch6/1 -> ref_sig_limit/1

== system gm_IP_Core_SS_Switch_and_PWM/PWM_and_Switching_Signal_Control/GenPWM/LimitPulseWidth6 ==
  note: Set pulse width in percent
  ref_sig : Inport  OutDataTypeStr=fixdt(1, 14, 12)  PortDimensions=1  SampleTime=1e-08
  min_pulse_width : Inport  Port=2  OutDataTypeStr=fixdt(1, 18, 16)  PortDimensions=1  SampleTime=1e-08
  Add : Sum  Inputs=+-  AccumDataTypeStr=fixdt(1, 19, 16)  OutDataTypeStr=fixdt(1, 18, 16)  SampleTime=1e-08
  Constant : Constant  OutDataTypeStr=fixdt(1, 18, 16)  SampleTime=1e-08
  Constant1 : Constant  Value=1.0099945068359375  OutDataTypeStr=fixdt(1, 18, 16)  SampleTime=1e-08
  Constant2 : Constant  Value=0  OutDataTypeStr=fixdt(1, 18, 16)  SampleTime=1e-08
  Logical Operator : Logic  Operator=OR  AllPortsSameDT=off  OutDataTypeStr=boolean  SampleTime=1e-08
  Relational Operator : RelationalOperator  Operator=>  OutDataTypeStr=boolean  SampleTime=1e-08  RndMeth=Nearest
  Relational Operator1 : RelationalOperator  Operator=<  OutDataTypeStr=boolean  SampleTime=1e-08  RndMeth=Nearest
  Saturation : Saturate  UpperLimit="fi(0,1,18,16,\"hex\",\"10000\")"  LowerLimit="fi(0,1,18,16,\"hex\",\"00000\")"  SampleTime=1e-08  OutDataTypeStr=fixdt(1, 18, 16)
  Switch1 : Switch  Criteria=u2 > Threshold  Threshold=double(0)  OutDataTypeStr=fixdt(1, 18, 16)  SampleTime=1e-08
  Switch6 : Switch  Criteria=u2 > Threshold  Threshold=double(0)  OutDataTypeStr=fixdt(1, 18, 16)  SampleTime=1e-08
  ref_sig_limit : Outport  SampleTime=1e-08  VectorParamsAs1DForOutWhenUnconnected=off
  wires:
  ref_sig/1 -> Switch6/3, Relational Operator1/1, Relational Operator/1
  min_pulse_width/1 -> Saturation/1, Add/2
  Add/1 -> Relational Operator/2
  Constant/1 -> Add/1
  Constant1/1 -> Switch1/3
  Constant2/1 -> Switch1/1
  Logical Operator/1 -> Switch6/2
  Relational Operator/1 -> Logical Operator/1
  Relational Operator1/1 -> Switch1/2, Logical Operator/2
  Saturation/1 -> Relational Operator1/2
  Switch1/1 -> Switch6/1
  Switch6/1 -> ref_sig_limit/1

== system gm_IP_Core_SS_Switch_and_PWM/PWM_and_Switching_Signal_Control/GenPWM/LimitPulseWidth7 ==
  note: Set pulse width in percent
  ref_sig : Inport  OutDataTypeStr=fixdt(1, 14, 12)  PortDimensions=1  SampleTime=1e-08
  min_pulse_width : Inport  Port=2  OutDataTypeStr=fixdt(1, 18, 16)  PortDimensions=1  SampleTime=1e-08
  Add : Sum  Inputs=+-  AccumDataTypeStr=fixdt(1, 19, 16)  OutDataTypeStr=fixdt(1, 18, 16)  SampleTime=1e-08
  Constant : Constant  OutDataTypeStr=fixdt(1, 18, 16)  SampleTime=1e-08
  Constant1 : Constant  Value=1.0099945068359375  OutDataTypeStr=fixdt(1, 18, 16)  SampleTime=1e-08
  Constant2 : Constant  Value=0  OutDataTypeStr=fixdt(1, 18, 16)  SampleTime=1e-08
  Logical Operator : Logic  Operator=OR  AllPortsSameDT=off  OutDataTypeStr=boolean  SampleTime=1e-08
  Relational Operator : RelationalOperator  Operator=>  OutDataTypeStr=boolean  SampleTime=1e-08  RndMeth=Nearest
  Relational Operator1 : RelationalOperator  Operator=<  OutDataTypeStr=boolean  SampleTime=1e-08  RndMeth=Nearest
  Saturation : Saturate  UpperLimit="fi(0,1,18,16,\"hex\",\"10000\")"  LowerLimit="fi(0,1,18,16,\"hex\",\"00000\")"  SampleTime=1e-08  OutDataTypeStr=fixdt(1, 18, 16)
  Switch1 : Switch  Criteria=u2 > Threshold  Threshold=double(0)  OutDataTypeStr=fixdt(1, 18, 16)  SampleTime=1e-08
  Switch6 : Switch  Criteria=u2 > Threshold  Threshold=double(0)  OutDataTypeStr=fixdt(1, 18, 16)  SampleTime=1e-08
  ref_sig_limit : Outport  SampleTime=1e-08  VectorParamsAs1DForOutWhenUnconnected=off
  wires:
  ref_sig/1 -> Switch6/3, Relational Operator1/1, Relational Operator/1
  min_pulse_width/1 -> Saturation/1, Add/2
  Add/1 -> Relational Operator/2
  Constant/1 -> Add/1
  Constant1/1 -> Switch1/3
  Constant2/1 -> Switch1/1
  Logical Operator/1 -> Switch6/2
  Relational Operator/1 -> Logical Operator/1
  Relational Operator1/1 -> Switch1/2, Logical Operator/2
  Saturation/1 -> Relational Operator1/2
  Switch1/1 -> Switch6/1
  Switch6/1 -> ref_sig_limit/1

== system gm_IP_Core_SS_Switch_and_PWM/PWM_and_Switching_Signal_Control/GenPWM/LimitPulseWidth8 ==
  note: Set pulse width in percent
  ref_sig : Inport  OutDataTypeStr=fixdt(1, 14, 12)  PortDimensions=1  SampleTime=1e-08
  min_pulse_width : Inport  Port=2  OutDataTypeStr=fixdt(1, 18, 16)  PortDimensions=1  SampleTime=1e-08
  Add : Sum  Inputs=+-  AccumDataTypeStr=fixdt(1, 19, 16)  OutDataTypeStr=fixdt(1, 18, 16)  SampleTime=1e-08
  Constant : Constant  OutDataTypeStr=fixdt(1, 18, 16)  SampleTime=1e-08
  Constant1 : Constant  Value=1.0099945068359375  OutDataTypeStr=fixdt(1, 18, 16)  SampleTime=1e-08
  Constant2 : Constant  Value=0  OutDataTypeStr=fixdt(1, 18, 16)  SampleTime=1e-08
  Logical Operator : Logic  Operator=OR  AllPortsSameDT=off  OutDataTypeStr=boolean  SampleTime=1e-08
  Relational Operator : RelationalOperator  Operator=>  OutDataTypeStr=boolean  SampleTime=1e-08  RndMeth=Nearest
  Relational Operator1 : RelationalOperator  Operator=<  OutDataTypeStr=boolean  SampleTime=1e-08  RndMeth=Nearest
  Saturation : Saturate  UpperLimit="fi(0,1,18,16,\"hex\",\"10000\")"  LowerLimit="fi(0,1,18,16,\"hex\",\"00000\")"  SampleTime=1e-08  OutDataTypeStr=fixdt(1, 18, 16)
  Switch1 : Switch  Criteria=u2 > Threshold  Threshold=double(0)  OutDataTypeStr=fixdt(1, 18, 16)  SampleTime=1e-08
  Switch6 : Switch  Criteria=u2 > Threshold  Threshold=double(0)  OutDataTypeStr=fixdt(1, 18, 16)  SampleTime=1e-08
  ref_sig_limit : Outport  SampleTime=1e-08  VectorParamsAs1DForOutWhenUnconnected=off
  wires:
  ref_sig/1 -> Switch6/3, Relational Operator1/1, Relational Operator/1
  min_pulse_width/1 -> Saturation/1, Add/2
  Add/1 -> Relational Operator/2
  Constant/1 -> Add/1
  Constant1/1 -> Switch1/3
  Constant2/1 -> Switch1/1
  Logical Operator/1 -> Switch6/2
  Relational Operator/1 -> Logical Operator/1
  Relational Operator1/1 -> Switch1/2, Logical Operator/2
  Saturation/1 -> Relational Operator1/2
  Switch1/1 -> Switch6/1
  Switch6/1 -> ref_sig_limit/1

== system gm_IP_Core_SS_Switch_and_PWM/PWM_and_Switching_Signal_Control/GenPWM/LimitPulseWidth9 ==
  note: Set pulse width in percent
  ref_sig : Inport  OutDataTypeStr=fixdt(1, 14, 12)  PortDimensions=1  SampleTime=1e-08
  min_pulse_width : Inport  Port=2  OutDataTypeStr=fixdt(1, 18, 16)  PortDimensions=1  SampleTime=1e-08
  Add : Sum  Inputs=+-  AccumDataTypeStr=fixdt(1, 19, 16)  OutDataTypeStr=fixdt(1, 18, 16)  SampleTime=1e-08
  Constant : Constant  OutDataTypeStr=fixdt(1, 18, 16)  SampleTime=1e-08
  Constant1 : Constant  Value=1.0099945068359375  OutDataTypeStr=fixdt(1, 18, 16)  SampleTime=1e-08
  Constant2 : Constant  Value=0  OutDataTypeStr=fixdt(1, 18, 16)  SampleTime=1e-08
  Logical Operator : Logic  Operator=OR  AllPortsSameDT=off  OutDataTypeStr=boolean  SampleTime=1e-08
  Relational Operator : RelationalOperator  Operator=>  OutDataTypeStr=boolean  SampleTime=1e-08  RndMeth=Nearest
  Relational Operator1 : RelationalOperator  Operator=<  OutDataTypeStr=boolean  SampleTime=1e-08  RndMeth=Nearest
  Saturation : Saturate  UpperLimit="fi(0,1,18,16,\"hex\",\"10000\")"  LowerLimit="fi(0,1,18,16,\"hex\",\"00000\")"  SampleTime=1e-08  OutDataTypeStr=fixdt(1, 18, 16)
  Switch1 : Switch  Criteria=u2 > Threshold  Threshold=double(0)  OutDataTypeStr=fixdt(1, 18, 16)  SampleTime=1e-08
  Switch6 : Switch  Criteria=u2 > Threshold  Threshold=double(0)  OutDataTypeStr=fixdt(1, 18, 16)  SampleTime=1e-08
  ref_sig_limit : Outport  SampleTime=1e-08  VectorParamsAs1DForOutWhenUnconnected=off
  wires:
  ref_sig/1 -> Switch6/3, Relational Operator1/1, Relational Operator/1
  min_pulse_width/1 -> Saturation/1, Add/2
  Add/1 -> Relational Operator/2
  Constant/1 -> Add/1
  Constant1/1 -> Switch1/3
  Constant2/1 -> Switch1/1
  Logical Operator/1 -> Switch6/2
  Relational Operator/1 -> Logical Operator/1
  Relational Operator1/1 -> Switch1/2, Logical Operator/2
  Saturation/1 -> Relational Operator1/2
  Switch1/1 -> Switch6/1
  Switch6/1 -> ref_sig_limit/1
